simulink model "TITO_TC_DE_2011"  (Simulink 7.7)
settings: Solver=ode45  StartTime=0.0  StopTime=100.0  RelTol=1e-3
libraries: simulink x2
settings Model: Creator=petr  LastModifiedBy=NICHOLAS ANG
settings OptimizationCC: InitFltsAndDblsToZero=on
settings DebuggingCC: FcnCallInpInsideContextMsg=Enable All
settings CodeAppCC: CustomSymbolStrType=$N$R$M_T
settings GRTTargetCC: TargetFunctionLibrary=C89/C90 (ANSI)  GeneratePreprocessorConditionals=Use local settings

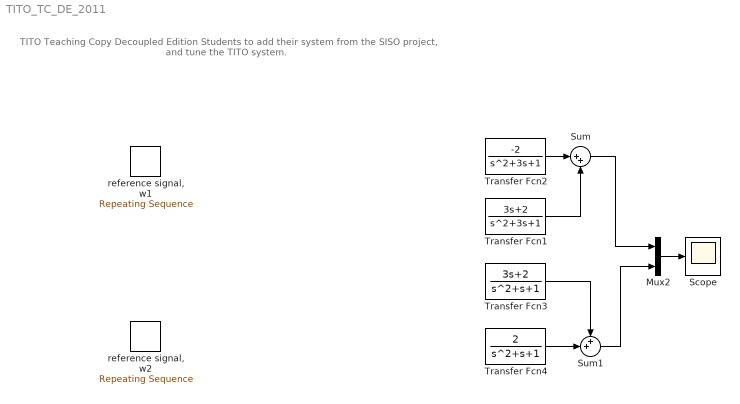
== system TITO_TC_DE_2011 ==
  note: TITO Teaching Copy Decoupled Edition
      |
      | Students to add their system from the SISO
      | project, and tune the TITO system.
  Mux2 : Mux  Inputs=2
  Scope : Scope
      settings: TimeRange=auto  MaxDataPoints=5000  SaveName=sd  YMin=-5  YMax=5  SampleTime=-1
  Sum : Sum  Inputs=|++
  Sum1 : Sum  Inputs=++|
  Transfer Fcn1 : TransferFcn  Numerator=[3 2]  Denominator=[1 3 1]
  Transfer Fcn2 : TransferFcn  Numerator=[-2]  Denominator=[1 3 1]
  Transfer Fcn3 : TransferFcn  Numerator=[3 2]  Denominator=[1 1 1]
  Transfer Fcn4 : TransferFcn  Numerator=[2]  Denominator=[1 1 1]
  "reference signal, w1" : simulink/Sources/Repeating Sequence  rep_seq_t=20*[0 0.4999 0.5 1.4999]  rep_seq_y=[1 1 2 2]
  "reference signal, w2" : simulink/Sources/Repeating Sequence  rep_seq_t=20*[0 0.9999 1.0 1.4999]  rep_seq_y=0.52*[1 1 2 2]
  wires:
  Transfer Fcn2/1 -> Sum/1
  Transfer Fcn1/1 -> Sum/2
  Transfer Fcn4/1 -> Sum1/2
  Transfer Fcn3/1 -> Sum1/1
  Sum/1 -> Mux2/1
  Sum1/1 -> Mux2/2
  Mux2/1 -> Scope/1
